simulink model "uc_faz_kompanzasyon"  (R2020b)
settings: Solver=VariableStepAuto  StartTime=0.0  StopTime=1  RelTol=1e-3  EnableMultiTasking=on
libraries: fl_lib x90, nesl_utility x45, powerlib_extras x15
settings Model: Creator=PC  LastModifiedBy=hilal
settings DataIOCC: ReturnWorkspaceOutputs=off
settings OptimizationCC: LifeSpan=inf
settings DebuggingCC: SFUnexpectedBacktrackingDiag=warning  SFNoUnconditionalDefaultTransitionDiag=warning  ArithmeticOperatorsInVariantConditions=warning
settings SFSimCC: SimUseLocalCustomCode=off  CustomCodeUndefinedFunction=UseInterfaceOnly
settings RTWCC: RTWUseLocalCustomCode=off
settings CodeAppCC: StateflowObjectComments=on
settings GRTTargetCC: TargetLangStandard=C89/C90 (ANSI)
settings ConfigComp: CovMetricSettings=dw  CovSaveCumulativeToWorkspaceVar=on  CovSaveSingleToWorkspaceVar=on  CovExternalEMLEnable=off
settings SimscapeCC: SimscapeNormalizeSystem=off

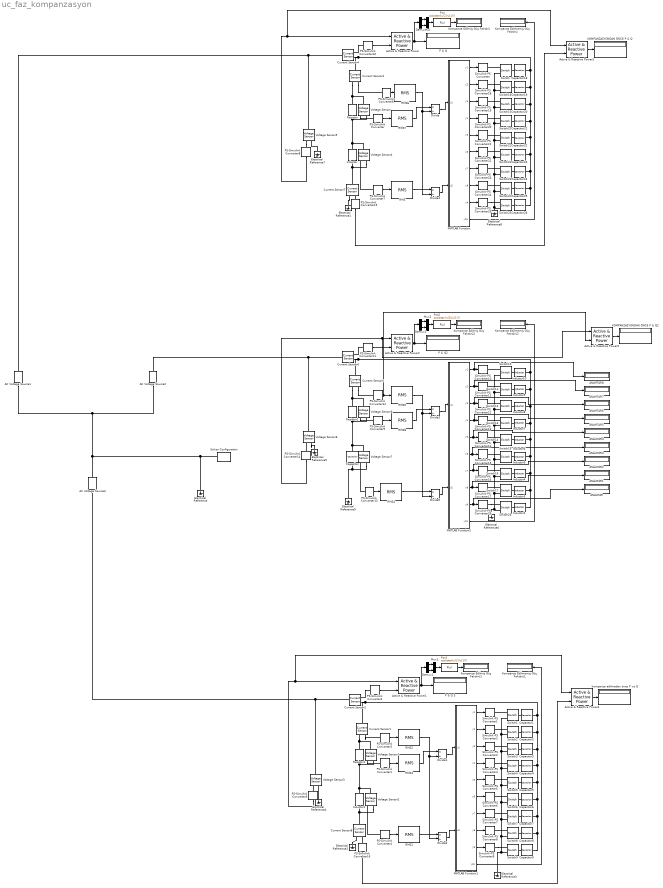
== system uc_faz_kompanzasyon ==
  AC Voltage Source1 : fl_lib/Electrical/Electrical Sources/AC Voltage Source  amp=200*sqrt(2) V  shift=0 rad  frequency=60 Hz  omega=50 Hz
  AC Voltage Source2 : fl_lib/Electrical/Electrical Sources/AC Voltage Source  amp=200*sqrt(2) V  shift=120 deg  frequency=60 Hz  omega=50 Hz
  AC Voltage Source3 : fl_lib/Electrical/Electrical Sources/AC Voltage Source  amp=200*sqrt(2) V  shift=240 deg  frequency=60 Hz  omega=50 Hz
  ANAHTAR{,1..8} (9 alike) : Display
  Active & Reactive Power{,1..5} (6 alike) : powerlib_extras/Measurements/Active & Reactive Power  f1=60
      settings: SourceProductBaseCode=PS
  Capacitor : fl_lib/Electrical/Electrical Elements/Capacitor  c=1/(20*2*pi*60) F  r=1e-6 Ohm  g=0 1/Ohm  i_specify=off  i_priority=None  i=0 A  i_nominal_specify=off  i_nominal_unit=A  i_nominal_value=1  v_specify=off  v_priority=None  v=0 V  v_nominal_specify=off  v_nominal_unit=V  v_nominal_value=1  vc_specify=off  vc_priority=High  vc=0 V  vc_nominal_specify=off  vc_nominal_unit=V  vc_nominal_value=1
  Capacitor1 : fl_lib/Electrical/Electrical Elements/Capacitor  c=5 uF  r=1e-6 Ohm  g=0 1/Ohm  i_specify=off  i_priority=None  i=0 A  i_nominal_specify=off  i_nominal_unit=A  i_nominal_value=1  v_specify=off  v_priority=None  v=0 V  v_nominal_specify=off  v_nominal_unit=V  v_nominal_value=1  vc_specify=off  vc_priority=High  vc=0 V  vc_nominal_specify=off  vc_nominal_unit=V  vc_nominal_value=1
  Capacitor18 : fl_lib/Electrical/Electrical Elements/Capacitor  c=6.319 uF  r=1e-6 Ohm  g=0 1/Ohm  i_specify=off  i_priority=None  i=0 A  i_nominal_specify=off  i_nominal_unit=A  i_nominal_value=1  v_specify=off  v_priority=None  v=0 V  v_nominal_specify=off  v_nominal_unit=V  v_nominal_value=1  vc_specify=off  vc_priority=High  vc=0 V  vc_nominal_specify=off  vc_nominal_unit=V  vc_nominal_value=1
  Capacitor19 : fl_lib/Electrical/Electrical Elements/Capacitor  c=15 uF  r=1e-6 Ohm  g=0 1/Ohm  i_specify=off  i_priority=None  i=0 A  i_nominal_specify=off  i_nominal_unit=A  i_nominal_value=1  v_specify=off  v_priority=None  v=0 V  v_nominal_specify=off  v_nominal_unit=V  v_nominal_value=1  vc_specify=off  vc_priority=High  vc=0 V  vc_nominal_specify=off  vc_nominal_unit=V  vc_nominal_value=1
  Capacitor2 : fl_lib/Electrical/Electrical Elements/Capacitor  c=15 uF  r=1e-6 Ohm  g=0 1/Ohm  i_specify=off  i_priority=None  i=0 A  i_nominal_specify=off  i_nominal_unit=A  i_nominal_value=1  v_specify=off  v_priority=None  v=0 V  v_nominal_specify=off  v_nominal_unit=V  v_nominal_value=1  vc_specify=off  vc_priority=High  vc=0 V  vc_nominal_specify=off  vc_nominal_unit=V  vc_nominal_value=1
  Capacitor20 : fl_lib/Electrical/Electrical Elements/Capacitor  c=24.6023 uF  r=1e-6 Ohm  g=0 1/Ohm  i_specify=off  i_priority=None  i=0 A  i_nominal_specify=off  i_nominal_unit=A  i_nominal_value=1  v_specify=off  v_priority=None  v=0 V  v_nominal_specify=off  v_nominal_unit=V  v_nominal_value=1  vc_specify=off  vc_priority=High  vc=0 V  vc_nominal_specify=off  vc_nominal_unit=V  vc_nominal_value=1
  Capacitor21 : fl_lib/Electrical/Electrical Elements/Capacitor  c=30.6 uF  r=1e-6 Ohm  g=0 1/Ohm  i_specify=off  i_priority=None  i=0 A  i_nominal_specify=off  i_nominal_unit=A  i_nominal_value=1  v_specify=off  v_priority=None  v=0 V  v_nominal_specify=off  v_nominal_unit=V  v_nominal_value=1  vc_specify=off  vc_priority=High  vc=0 V  vc_nominal_specify=off  vc_nominal_unit=V  vc_nominal_value=1
  Capacitor22 : fl_lib/Electrical/Electrical Elements/Capacitor  c=44.59 uF  r=1e-6 Ohm  g=0 1/Ohm  i_specify=off  i_priority=None  i=0 A  i_nominal_specify=off  i_nominal_unit=A  i_nominal_value=1  v_specify=off  v_priority=None  v=0 V  v_nominal_specify=off  v_nominal_unit=V  v_nominal_value=1  vc_specify=off  vc_priority=High  vc=0 V  vc_nominal_specify=off  vc_nominal_unit=V  vc_nominal_value=1
  Capacitor23 : fl_lib/Electrical/Electrical Elements/Capacitor  c=53.575 uF  r=1e-6 Ohm  g=0 1/Ohm  i_specify=off  i_priority=None  i=0 A  i_nominal_specify=off  i_nominal_unit=A  i_nominal_value=1  v_specify=off  v_priority=None  v=0 V  v_nominal_specify=off  v_nominal_unit=V  v_nominal_value=1  vc_specify=off  vc_priority=High  vc=0 V  vc_nominal_specify=off  vc_nominal_unit=V  vc_nominal_value=1
  Capacitor24 : fl_lib/Electrical/Electrical Elements/Capacitor  c=62.234 uF  r=1e-6 Ohm  g=0 1/Ohm  i_specify=off  i_priority=None  i=0 A  i_nominal_specify=off  i_nominal_unit=A  i_nominal_value=1  v_specify=off  v_priority=None  v=0 V  v_nominal_specify=off  v_nominal_unit=V  v_nominal_value=1  vc_specify=off  vc_priority=High  vc=0 V  vc_nominal_specify=off  vc_nominal_unit=V  vc_nominal_value=1
  Capacitor25 : fl_lib/Electrical/Electrical Elements/Capacitor  c=70.9489 uF  r=1e-6 Ohm  g=0 1/Ohm  i_specify=off  i_priority=None  i=0 A  i_nominal_specify=off  i_nominal_unit=A  i_nominal_value=1  v_specify=off  v_priority=None  v=0 V  v_nominal_specify=off  v_nominal_unit=V  v_nominal_value=1  vc_specify=off  vc_priority=High  vc=0 V  vc_nominal_specify=off  vc_nominal_unit=V  vc_nominal_value=1
  Capacitor26 : fl_lib/Electrical/Electrical Elements/Capacitor  c=78.304 uF  r=1e-6 Ohm  g=0 1/Ohm  i_specify=off  i_priority=None  i=0 A  i_nominal_specify=off  i_nominal_unit=A  i_nominal_value=1  v_specify=off  v_priority=None  v=0 V  v_nominal_specify=off  v_nominal_unit=V  v_nominal_value=1  vc_specify=off  vc_priority=High  vc=0 V  vc_nominal_specify=off  vc_nominal_unit=V  vc_nominal_value=1
  Capacitor3 : fl_lib/Electrical/Electrical Elements/Capacitor  c=24.6023 uF  r=1e-6 Ohm  g=0 1/Ohm  i_specify=off  i_priority=None  i=0 A  i_nominal_specify=off  i_nominal_unit=A  i_nominal_value=1  v_specify=off  v_priority=None  v=0 V  v_nominal_specify=off  v_nominal_unit=V  v_nominal_value=1  vc_specify=off  vc_priority=High  vc=0 V  vc_nominal_specify=off  vc_nominal_unit=V  vc_nominal_value=1
  Capacitor4 : fl_lib/Electrical/Electrical Elements/Capacitor  c=30.6 uF  r=1e-6 Ohm  g=0 1/Ohm  i_specify=off  i_priority=None  i=0 A  i_nominal_specify=off  i_nominal_unit=A  i_nominal_value=1  v_specify=off  v_priority=None  v=0 V  v_nominal_specify=off  v_nominal_unit=V  v_nominal_value=1  vc_specify=off  vc_priority=High  vc=0 V  vc_nominal_specify=off  vc_nominal_unit=V  vc_nominal_value=1
  Capacitor5 : fl_lib/Electrical/Electrical Elements/Capacitor  c=44.59 uF  r=1e-6 Ohm  g=0 1/Ohm  i_specify=off  i_priority=None  i=0 A  i_nominal_specify=off  i_nominal_unit=A  i_nominal_value=1  v_specify=off  v_priority=None  v=0 V  v_nominal_specify=off  v_nominal_unit=V  v_nominal_value=1  vc_specify=off  vc_priority=High  vc=0 V  vc_nominal_specify=off  vc_nominal_unit=V  vc_nominal_value=1
  Capacitor6 : fl_lib/Electrical/Electrical Elements/Capacitor  c=53.575 uF  r=1e-6 Ohm  g=0 1/Ohm  i_specify=off  i_priority=None  i=0 A  i_nominal_specify=off  i_nominal_unit=A  i_nominal_value=1  v_specify=off  v_priority=None  v=0 V  v_nominal_specify=off  v_nominal_unit=V  v_nominal_value=1  vc_specify=off  vc_priority=High  vc=0 V  vc_nominal_specify=off  vc_nominal_unit=V  vc_nominal_value=1
  Capacitor7 : fl_lib/Electrical/Electrical Elements/Capacitor  c=62.234 uF  r=1e-6 Ohm  g=0 1/Ohm  i_specify=off  i_priority=None  i=0 A  i_nominal_specify=off  i_nominal_unit=A  i_nominal_value=1  v_specify=off  v_priority=None  v=0 V  v_nominal_specify=off  v_nominal_unit=V  v_nominal_value=1  vc_specify=off  vc_priority=High  vc=0 V  vc_nominal_specify=off  vc_nominal_unit=V  vc_nominal_value=1
  Capacitor8 : fl_lib/Electrical/Electrical Elements/Capacitor  c=70.9489 uF  r=1e-6 Ohm  g=0 1/Ohm  i_specify=off  i_priority=None  i=0 A  i_nominal_specify=off  i_nominal_unit=A  i_nominal_value=1  v_specify=off  v_priority=None  v=0 V  v_nominal_specify=off  v_nominal_unit=V  v_nominal_value=1  vc_specify=off  vc_priority=High  vc=0 V  vc_nominal_specify=off  vc_nominal_unit=V  vc_nominal_value=1
  Capacitor9 : fl_lib/Electrical/Electrical Elements/Capacitor  c=78.304 uF  r=1e-6 Ohm  g=0 1/Ohm  i_specify=off  i_priority=None  i=0 A  i_nominal_specify=off  i_nominal_unit=A  i_nominal_value=1  v_specify=off  v_priority=None  v=0 V  v_nominal_specify=off  v_nominal_unit=V  v_nominal_value=1  vc_specify=off  vc_priority=High  vc=0 V  vc_nominal_specify=off  vc_nominal_unit=V  vc_nominal_value=1
  Current Sensor{1..8} (8 alike) : fl_lib/Electrical/Electrical Sensors/Current Sensor
  Demux : Demux  Outputs=2
  Demux1 : Demux  Outputs=2
  Demux2 : Demux  Outputs=2
  Divide{,1..5} (6 alike) : Product  Inputs=*/
  Electrical Reference{,1..9} (10 alike) : fl_lib/Electrical/Electrical Elements/Electrical Reference
  Fcn : Fcn  Expr=cos(atan(u(2)/u(1)))
  Fcn1 : Fcn  Expr=cos(atan(u(2)/u(1)))
  Fcn2 : Fcn  Expr=cos(atan(u(2)/u(1)))
  Inductor : fl_lib/Electrical/Electrical Elements/Inductor  l=20/(2*pi*60) H  r=0 Ohm  g=1e-9 1/Ohm  i_specify=off  i_priority=None  i=0 A  i_nominal_specify=off  i_nominal_unit=A  i_nominal_value=1  v_specify=off  v_priority=None  v=0 V  v_nominal_specify=off  v_nominal_unit=V  v_nominal_value=1  i_L_specify=off  i_L_priority=High  i_L=0 A  i_L_nominal_specify=off  i_L_nominal_unit=A  i_L_nominal_value=1
  Inductor1 : fl_lib/Electrical/Electrical Elements/Inductor  l=20/(2*pi*60) H  r=0 Ohm  g=1e-9 1/Ohm  i_specify=off  i_priority=None  i=0 A  i_nominal_specify=off  i_nominal_unit=A  i_nominal_value=1  v_specify=off  v_priority=None  v=0 V  v_nominal_specify=off  v_nominal_unit=V  v_nominal_value=1  i_L_specify=off  i_L_priority=High  i_L=0 A  i_L_nominal_specify=off  i_L_nominal_unit=A  i_L_nominal_value=1
  Inductor10 : fl_lib/Electrical/Electrical Elements/Inductor  l=1234 mH  r=0 Ohm  g=1e-9 1/Ohm  i_specify=off  i_priority=None  i=0 A  i_nominal_specify=off  i_nominal_unit=A  i_nominal_value=1  v_specify=off  v_priority=None  v=0 V  v_nominal_specify=off  v_nominal_unit=V  v_nominal_value=1  i_L_specify=off  i_L_priority=High  i_L=0 A  i_L_nominal_specify=off  i_L_nominal_unit=A  i_L_nominal_value=1
  Inductor2 : fl_lib/Electrical/Electrical Elements/Inductor  l=89.5 mH  r=0 Ohm  g=1e-9 1/Ohm  i_specify=off  i_priority=None  i=0 A  i_nominal_specify=off  i_nominal_unit=A  i_nominal_value=1  v_specify=off  v_priority=None  v=0 V  v_nominal_specify=off  v_nominal_unit=V  v_nominal_value=1  i_L_specify=off  i_L_priority=High  i_L=0 A  i_L_nominal_specify=off  i_L_nominal_unit=A  i_L_nominal_value=1
  Inductor3 : fl_lib/Electrical/Electrical Elements/Inductor  l=99 mH  r=0 Ohm  g=1e-9 1/Ohm  i_specify=off  i_priority=None  i=0 A  i_nominal_specify=off  i_nominal_unit=A  i_nominal_value=1  v_specify=off  v_priority=None  v=0 V  v_nominal_specify=off  v_nominal_unit=V  v_nominal_value=1  i_L_specify=off  i_L_priority=High  i_L=0 A  i_L_nominal_specify=off  i_L_nominal_unit=A  i_L_nominal_value=1
  Inductor4 : fl_lib/Electrical/Electrical Elements/Inductor  l=109.9 mH  r=0 Ohm  g=1e-9 1/Ohm  i_specify=off  i_priority=None  i=0 A  i_nominal_specify=off  i_nominal_unit=A  i_nominal_value=1  v_specify=off  v_priority=None  v=0 V  v_nominal_specify=off  v_nominal_unit=V  v_nominal_value=1  i_L_specify=off  i_L_priority=High  i_L=0 A  i_L_nominal_specify=off  i_L_nominal_unit=A  i_L_nominal_value=1
  Inductor5 : fl_lib/Electrical/Electrical Elements/Inductor  l=136 mH  r=0 Ohm  g=1e-9 1/Ohm  i_specify=off  i_priority=None  i=0 A  i_nominal_specify=off  i_nominal_unit=A  i_nominal_value=1  v_specify=off  v_priority=None  v=0 V  v_nominal_specify=off  v_nominal_unit=V  v_nominal_value=1  i_L_specify=off  i_L_priority=High  i_L=0 A  i_L_nominal_specify=off  i_L_nominal_unit=A  i_L_nominal_value=1
  Inductor6 : fl_lib/Electrical/Electrical Elements/Inductor  l=158 mH  r=0 Ohm  g=1e-9 1/Ohm  i_specify=off  i_priority=None  i=0 A  i_nominal_specify=off  i_nominal_unit=A  i_nominal_value=1  v_specify=off  v_priority=None  v=0 V  v_nominal_specify=off  v_nominal_unit=V  v_nominal_value=1  i_L_specify=off  i_L_priority=High  i_L=0 A  i_L_nominal_specify=off  i_L_nominal_unit=A  i_L_nominal_value=1
  Inductor7 : fl_lib/Electrical/Electrical Elements/Inductor  l=210 mH  r=0 Ohm  g=1e-9 1/Ohm  i_specify=off  i_priority=None  i=0 A  i_nominal_specify=off  i_nominal_unit=A  i_nominal_value=1  v_specify=off  v_priority=None  v=0 V  v_nominal_specify=off  v_nominal_unit=V  v_nominal_value=1  i_L_specify=off  i_L_priority=High  i_L=0 A  i_L_nominal_specify=off  i_L_nominal_unit=A  i_L_nominal_value=1
  Inductor8 : fl_lib/Electrical/Electrical Elements/Inductor  l=269 mH  r=0 Ohm  g=1e-9 1/Ohm  i_specify=off  i_priority=None  i=0 A  i_nominal_specify=off  i_nominal_unit=A  i_nominal_value=1  v_specify=off  v_priority=None  v=0 V  v_nominal_specify=off  v_nominal_unit=V  v_nominal_value=1  i_L_specify=off  i_L_priority=High  i_L=0 A  i_L_nominal_specify=off  i_L_nominal_unit=A  i_L_nominal_value=1
  Inductor9 : fl_lib/Electrical/Electrical Elements/Inductor  l=508 mH  r=0 Ohm  g=1e-9 1/Ohm  i_specify=off  i_priority=None  i=0 A  i_nominal_specify=off  i_nominal_unit=A  i_nominal_value=1  v_specify=off  v_priority=None  v=0 V  v_nominal_specify=off  v_nominal_unit=V  v_nominal_value=1  i_L_specify=off  i_L_priority=High  i_L=0 A  i_L_nominal_specify=off  i_L_nominal_unit=A  i_L_nominal_value=1
  KOMPANZASYONDAN ÖNCE P & Q : Display
  KOMPANZASYONDAN ÖNCE P & Q2 : Display
  Kompanze Edilmemiş Güç Faktörü : Display
  Kompanze Edilmemiş Güç Faktörü1 : Display
  Kompanze Edilmemiş Güç Faktörü2 : Display
  Kompanze Edilmiş Güç Faktörü : Display
  Kompanze Edilmiş Güç Faktörü1 : Display
  Kompanze Edilmiş Güç Faktörü2 : Display
  MATLAB Function : MATLAB Function  TreatAsAtomicUnit=on
  MATLAB Function1 : MATLAB Function  TreatAsAtomicUnit=on
  MATLAB Function2 : MATLAB Function  TreatAsAtomicUnit=on
  Mux : Mux  Inputs=2
  Mux1 : Mux  Inputs=2
  Mux2 : Mux  Inputs=2
  P & Q : Display
  P & Q 3 : Display
  P & Q2 : Display
  PS-Simulink Converter{,1..16} (17 alike) : nesl_utility/PS-Simulink Converter  PhysicalDomain=network_engine_domain  SubClassName=ps_output  LeftPortType=input  RightPortType=output  PseudoPeriodic=off  Frequencies=[]  Unit=1  AffineConversion=off
  RMS{,1..8} (9 alike) : powerlib_extras/Measurements/RMS  f1=60
      settings: SourceProductBaseCode=PS
  Resistor : fl_lib/Electrical/Electrical Elements/Resistor  R=45 Ohm  i_specify=off  i_priority=None  i=0 A  i_nominal_specify=off  i_nominal_unit=A  i_nominal_value=1  v_specify=off  v_priority=None  v=0 V  v_nominal_specify=off  v_nominal_unit=V  v_nominal_value=1
  Resistor1 : fl_lib/Electrical/Electrical Elements/Resistor  R=13.5 Ohm  i_specify=off  i_priority=None  i=0 A  i_nominal_specify=off  i_nominal_unit=A  i_nominal_value=1  v_specify=off  v_priority=None  v=0 V  v_nominal_specify=off  v_nominal_unit=V  v_nominal_value=1
  Resistor2 : fl_lib/Electrical/Electrical Elements/Resistor  R=20 Ohm  i_specify=off  i_priority=None  i=0 A  i_nominal_specify=off  i_nominal_unit=A  i_nominal_value=1  v_specify=off  v_priority=None  v=0 V  v_nominal_specify=off  v_nominal_unit=V  v_nominal_value=1
  Simulink-PS Converter{,1..26} (27 alike) : nesl_utility/Simulink-PS Converter  PhysicalDomain=network_engine_domain  SubClassName=ps_input  LeftPortType=input  RightPortType=output  PseudoPeriodic=off  Frequencies=[]  NoiseDistribution=none  NoiseParameters=[]  Unit=1  AffineConversion=off  FilteringAndDerivatives=zero  SimscapeFilterOrder=1  InputFilterTimeConstant=0.001  UdotUserProvided=1
  Solver Configuration : nesl_utility/Solver Configuration  PhysicalDomain=network_engine_domain  SubClassName=solver  LeftPortType=input  RightPortType=generic  Tones=[]  Harmonics=[]  SimulateNoise=off  Profile=off  UseLocalSampling=off  EnableSwitchedLinearOptims=on  FrequencyDomain=off  UseCCode=off  RelTol=0.001  AbsTol=1e-06  MinStep=1e-09  ToWorkspace=off  RevertToSquareIcSolve=off  NumHomotopyIterations=100  PhasorMode=off  PhasorModeNumHarmonics=1  DoDC=on  ResidualTolerance=1e-9  UseLocalSolver=off  LocalSolverChoice=NE_BACKWARD_EULER_ADVANCER  LocalSolverSampleTime=.001  DoFixedCost=off  MaxNonlinIter=3  MaxModeIter=2  ComputeImpulses=off  ImpulseIterations=2  LinearAlgebra=Sparse  EquationFormulation=NE_TIME_EF  DelaysMemoryBudget=1024  AutomaticFiltering=on  FilteringTimeConstant=0.001  PartitionStorageMethod=AS_NEEDED  PartitionMemoryBudget=1024  PartitionMethod=FAST
  Switch{,1..26} (27 alike) : fl_lib/Electrical/Electrical Elements/Switch  R_closed=0.01 Ohm  G_open=1e-8 1/Ohm  Threshold=0  i_specify=off  i_priority=None  i=0 A  i_nominal_specify=off  i_nominal_unit=A  i_nominal_value=1  v_specify=off  v_priority=None  v=0 V  v_nominal_specify=off  v_nominal_unit=V  v_nominal_value=1
  Voltage Sensor{,1..8} (9 alike) : fl_lib/Electrical/Electrical Sensors/Voltage Sensor
  kompanze edilmeden önce P ve Q : Display
  wires:
  MATLAB Function/1(y1) -> Simulink-PS Converter/1
  MATLAB Function/3(y3) -> Simulink-PS Converter19/1
  MATLAB Function/5(y5) -> Simulink-PS Converter21/1
  MATLAB Function/7(y7) -> Simulink-PS Converter23/1
  MATLAB Function/8(y8) -> Simulink-PS Converter24/1
  MATLAB Function/6(y6) -> Simulink-PS Converter22/1
  Divide/1 -> MATLAB Function/1(u1)
  MATLAB Function/9(y9) -> Simulink-PS Converter25/1
  PS-Simulink Converter6/1 -> RMS6/1
  PS-Simulink Converter/1 -> RMS7/1
  PS-Simulink Converter7/1 -> RMS/1
  RMS/1 -> Divide4/1
  RMS6/1 -> Divide/2, Divide4/2
  RMS7/1 -> Divide/1
  Active & Reactive Power/1 -> P & Q/1, Demux/1
  Divide4/1 -> MATLAB Function/2(u2)
  PS-Simulink Converter10/1 -> Active & Reactive Power/2
  MATLAB Function/10(y10) -> Kompanze Edilmemiş Güç Faktörü/1
  Demux/1 -> Mux/1
  Demux/2 -> Mux/2
  Mux/1 -> Fcn/1
  Fcn/1 -> Kompanze Edilmiş Güç Faktörü/1
  MATLAB Function1/1(y1) -> Simulink-PS Converter1/1
  MATLAB Function1/2(y2) -> Simulink-PS Converter2/1
  MATLAB Function1/3(y3) -> Simulink-PS Converter3/1
  MATLAB Function1/4(y4) -> Simulink-PS Converter4/1
  MATLAB Function1/5(y5) -> Simulink-PS Converter5/1
  MATLAB Function1/7(y7) -> Simulink-PS Converter7/1
  MATLAB Function1/8(y8) -> Simulink-PS Converter8/1
  MATLAB Function1/6(y6) -> Simulink-PS Converter6/1
  Divide1/1 -> MATLAB Function1/1(u1)
  PS-Simulink Converter3/1 -> RMS2/1
  PS-Simulink Converter1/1 -> RMS3/1
  PS-Simulink Converter4/1 -> RMS1/1
  RMS1/1 -> Divide2/1
  RMS2/1 -> Divide1/2, Divide2/2
  RMS3/1 -> Divide1/1
  Active & Reactive Power1/1 -> P & Q 3/1, Demux1/1
  PS-Simulink Converter5/1 -> Active & Reactive Power4/1, Active & Reactive Power1/1
  Divide2/1 -> MATLAB Function1/2(u2)
  PS-Simulink Converter2/1 -> Active & Reactive Power1/2
  MATLAB Function1/10(y10) -> Kompanze Edilmemiş Güç Faktörü1/1
  Demux1/1 -> Mux1/1
  Demux1/2 -> Mux1/2
  Mux1/1 -> Fcn1/1
  Fcn1/1 -> Kompanze Edilmiş Güç Faktörü1/1
  MATLAB Function2/1(y1) -> ANAHTAR8/1, Simulink-PS Converter10/1
  MATLAB Function2/2(y2) -> ANAHTAR7/1, Simulink-PS Converter11/1
  MATLAB Function2/3(y3) -> ANAHTAR6/1, Simulink-PS Converter12/1
  MATLAB Function2/4(y4) -> ANAHTAR5/1, Simulink-PS Converter13/1
  MATLAB Function2/5(y5) -> ANAHTAR4/1, Simulink-PS Converter14/1
  MATLAB Function2/7(y7) -> ANAHTAR2/1, Simulink-PS Converter16/1
  MATLAB Function2/8(y8) -> ANAHTAR1/1, Simulink-PS Converter17/1
  MATLAB Function2/6(y6) -> ANAHTAR3/1, Simulink-PS Converter15/1
  Divide3/1 -> MATLAB Function2/1(u1)
  MATLAB Function2/9(y9) -> ANAHTAR/1, Simulink-PS Converter26/1
  PS-Simulink Converter12/1 -> Active & Reactive Power5/2, RMS5/1
  PS-Simulink Converter9/1 -> RMS8/1
  PS-Simulink Converter13/1 -> RMS4/1
  RMS5/1 -> Divide3/2, Divide5/2
  RMS8/1 -> Divide3/1
  Active & Reactive Power2/1 -> P & Q2/1, Demux2/1
  PS-Simulink Converter14/1 -> Active & Reactive Power5/1, Active & Reactive Power2/1
  Divide5/1 -> MATLAB Function2/2(u2)
  PS-Simulink Converter11/1 -> Active & Reactive Power2/2
  MATLAB Function2/10(y10) -> Kompanze Edilmemiş Güç Faktörü2/1
  Demux2/1 -> Mux2/1
  Demux2/2 -> Mux2/2
  Mux2/1 -> Fcn2/1
  Fcn2/1 -> Kompanze Edilmiş Güç Faktörü2/1
  RMS4/1 -> Divide5/1
  MATLAB Function/2(y2) -> Simulink-PS Converter18/1
  MATLAB Function/4(y4) -> Simulink-PS Converter20/1
  Active & Reactive Power3/1 -> KOMPANZASYONDAN ÖNCE P & Q/1
  PS-Simulink Converter8/1 -> Active & Reactive Power3/1, Active & Reactive Power/1
  PS-Simulink Converter15/1 -> Active & Reactive Power3/2
  Active & Reactive Power4/1 -> kompanze edilmeden önce P ve Q/1
  PS-Simulink Converter16/1 -> Active & Reactive Power4/2
  MATLAB Function1/9(y9) -> Simulink-PS Converter9/1
  Active & Reactive Power5/1 -> KOMPANZASYONDAN ÖNCE P & Q2/1
  connections:
  Capacitor21/RConn1 -- Current Sensor3/LConn1 -- Current Sensor4/RConn2 -- Capacitor18/RConn1 -- Capacitor19/RConn1 -- Capacitor20/RConn1 -- Capacitor26/RConn1 -- Capacitor25/RConn1 -- Capacitor24/RConn1 -- Capacitor23/RConn1 -- Capacitor22/RConn1
  Resistor/RConn1 -- Voltage Sensor/RConn2 -- Voltage Sensor4/LConn1 -- Inductor/LConn1
  Voltage Sensor/LConn1 -- Resistor/LConn1 -- Current Sensor3/RConn2
  Current Sensor4/LConn1 -- Voltage Sensor5/LConn1 -- AC Voltage Source1/LConn1
  Capacitor19/LConn1 -- Switch18/LConn1
  Capacitor20/LConn1 -- Switch19/LConn1
  Capacitor21/LConn1 -- Switch20/LConn1
  Switch23/RConn1 -- Simulink-PS Converter23/RConn1
  Capacitor24/LConn1 -- Switch23/LConn1
  Voltage Sensor/RConn1 -- PS-Simulink Converter/LConn1
  Capacitor25/LConn1 -- Switch24/LConn1
  Simulink-PS Converter25/RConn1 -- Switch25/RConn1
  Switch20/RConn1 -- Simulink-PS Converter20/RConn1
  Capacitor26/LConn1 -- Switch25/LConn1
  Switch19/RConn1 -- Simulink-PS Converter19/RConn1
  Switch22/RConn1 -- Simulink-PS Converter22/RConn1
  Capacitor18/LConn1 -- Switch/LConn1
  Switch/RConn1 -- Simulink-PS Converter/RConn1
  Capacitor22/LConn1 -- Switch21/LConn1
  Capacitor23/LConn1 -- Switch22/LConn1
  Voltage Sensor5/RConn1 -- PS-Simulink Converter8/LConn1
  Switch18/RConn1 -- Simulink-PS Converter18/RConn1
  PS-Simulink Converter7/LConn1 -- Voltage Sensor4/RConn1
  Current Sensor4/RConn1 -- PS-Simulink Converter10/LConn1
  Switch21/RConn1 -- Simulink-PS Converter21/RConn1
  Switch24/RConn1 -- Simulink-PS Converter24/RConn1
  Capacitor4/RConn1 -- Current Sensor1/LConn1 -- Current Sensor2/RConn2 -- Capacitor1/RConn1 -- Capacitor2/RConn1 -- Capacitor3/RConn1 -- Capacitor5/RConn1 -- Capacitor6/RConn1 -- Capacitor7/RConn1 -- Capacitor9/RConn1 -- Capacitor8/RConn1
  AC Voltage Source2/RConn1 -- AC Voltage Source1/RConn1 -- Electrical Reference/LConn1 -- Solver Configuration/RConn1 -- AC Voltage Source3/RConn1
  Inductor1/LConn1 -- Voltage Sensor2/LConn1 -- Voltage Sensor1/RConn2 -- Resistor1/RConn1
  Voltage Sensor1/LConn1 -- Resistor1/LConn1 -- Current Sensor1/RConn2
  Current Sensor2/LConn1 -- Voltage Sensor3/LConn1 -- AC Voltage Source3/LConn1
  Voltage Sensor1/RConn1 -- PS-Simulink Converter1/LConn1
  Capacitor2/LConn1 -- Switch2/LConn1
  Capacitor4/LConn1 -- Switch4/LConn1
  Current Sensor1/RConn1 -- PS-Simulink Converter3/LConn1
  PS-Simulink Converter4/LConn1 -- Voltage Sensor2/RConn1
  Capacitor8/LConn1 -- Switch8/LConn1
  Capacitor6/LConn1 -- Switch6/LConn1
  Switch3/RConn1 -- Simulink-PS Converter3/RConn1
  Switch6/RConn1 -- Simulink-PS Converter6/RConn1
  Switch1/RConn1 -- Simulink-PS Converter1/RConn1
  Switch5/RConn1 -- Simulink-PS Converter5/RConn1
  Capacitor9/LConn1 -- Switch9/LConn1
  Switch8/RConn1 -- Simulink-PS Converter8/RConn1
  Capacitor7/LConn1 -- Switch7/LConn1
  Simulink-PS Converter9/RConn1 -- Switch9/RConn1
  Switch7/RConn1 -- Simulink-PS Converter7/RConn1
  Capacitor3/LConn1 -- Switch3/LConn1
  Capacitor1/LConn1 -- Switch1/LConn1
  Switch4/RConn1 -- Simulink-PS Converter4/RConn1
  Current Sensor2/RConn1 -- PS-Simulink Converter2/LConn1
  Switch2/RConn1 -- Simulink-PS Converter2/RConn1
  Capacitor5/LConn1 -- Switch5/LConn1
  Inductor7/RConn1 -- Inductor6/RConn1 -- Inductor5/RConn1 -- Inductor4/RConn1 -- Inductor3/RConn1 -- Inductor2/RConn1 -- Inductor9/RConn1 -- Inductor10/RConn1 -- Current Sensor5/LConn1 -- Current Sensor6/RConn2 -- Inductor8/RConn1
  Voltage Sensor7/LConn1 -- Capacitor/LConn1 -- Voltage Sensor6/RConn2 -- Resistor2/RConn1
  Voltage Sensor6/LConn1 -- Resistor2/LConn1 -- Current Sensor5/RConn2
  Inductor4/LConn1 -- Switch16/LConn1
  Switch13/RConn1 -- Simulink-PS Converter13/RConn1
  Inductor10/LConn1 -- Switch10/LConn1
  Switch11/RConn1 -- Simulink-PS Converter11/RConn1
  Switch10/RConn1 -- Simulink-PS Converter10/RConn1
  Switch12/RConn1 -- Simulink-PS Converter12/RConn1
  Voltage Sensor6/RConn1 -- PS-Simulink Converter9/LConn1
  Inductor9/LConn1 -- Switch11/LConn1
  Switch14/RConn1 -- Simulink-PS Converter14/RConn1
  Current Sensor6/RConn1 -- PS-Simulink Converter11/LConn1
  Inductor8/LConn1 -- Switch12/LConn1
  Inductor3/LConn1 -- Switch17/LConn1
  Current Sensor5/RConn1 -- PS-Simulink Converter12/LConn1
  Inductor2/LConn1 -- Switch26/LConn1
  Switch15/RConn1 -- Simulink-PS Converter15/RConn1
  Switch16/RConn1 -- Simulink-PS Converter16/RConn1
  Inductor7/LConn1 -- Switch13/LConn1
  Inductor5/LConn1 -- Switch15/LConn1
  Inductor6/LConn1 -- Switch14/LConn1
  Switch17/RConn1 -- Simulink-PS Converter17/RConn1
  Simulink-PS Converter26/RConn1 -- Switch26/RConn1
  PS-Simulink Converter13/LConn1 -- Voltage Sensor7/RConn1
  PS-Simulink Converter14/LConn1 -- Voltage Sensor8/RConn1
  AC Voltage Source2/LConn1 -- Current Sensor6/LConn1 -- Voltage Sensor8/LConn1
  Current Sensor3/RConn1 -- PS-Simulink Converter6/LConn1
  Voltage Sensor4/RConn2 -- Inductor/RConn1 -- Current Sensor7/LConn1
  PS-Simulink Converter15/LConn1 -- Current Sensor7/RConn1
  Current Sensor7/RConn2 -- Electrical Reference1/LConn1
  Voltage Sensor2/RConn2 -- Inductor1/RConn1 -- Current Sensor8/LConn1
  Current Sensor8/RConn2 -- Electrical Reference2/LConn1
  PS-Simulink Converter16/LConn1 -- Current Sensor8/RConn1
  PS-Simulink Converter5/LConn1 -- Voltage Sensor3/RConn1
  Switch9/RConn2 -- Electrical Reference3/LConn1 -- Switch4/RConn2 -- Switch3/RConn2 -- Switch1/RConn2 -- Switch2/RConn2 -- Switch5/RConn2 -- Switch6/RConn2 -- Switch7/RConn2 -- Switch8/RConn2
  Electrical Reference4/LConn1 -- Voltage Sensor3/RConn2
  Voltage Sensor8/RConn2 -- Electrical Reference5/LConn1
  Switch17/RConn2 -- Electrical Reference6/LConn1 -- Switch26/RConn2 -- Switch13/RConn2 -- Switch12/RConn2 -- Switch10/RConn2 -- Switch11/RConn2 -- Switch14/RConn2 -- Switch15/RConn2 -- Switch16/RConn2
  Electrical Reference7/LConn1 -- Voltage Sensor5/RConn2
  Switch23/RConn2 -- Electrical Reference8/LConn1 -- Switch25/RConn2 -- Switch24/RConn2 -- Switch20/RConn2 -- Switch19/RConn2 -- Switch/RConn2 -- Switch18/RConn2 -- Switch21/RConn2 -- Switch22/RConn2
  Voltage Sensor7/RConn2 -- Electrical Reference9/LConn1 -- Capacitor/RConn1

== matlab function uc_faz_kompanzasyon/MATLAB Function1 ==
  data: u1 input; y1 output; u2 input; y2 output; y3 output; y4 output; y5 output; y6 output; y7 output; y8 output; y9 output; y10 output
function [y1,y2,y3,y4,y5,y6,y7,y8,y9,y10] = fcn(u1,u2)
R=u1;% 1. değişken
L=u2;% 1. değişken

V=200;

I=200/(R+i*L);
Iconj=conj(I);

S=V*Iconj;
P=real(S);
Q=imag(S);

teta=angle(S);
pf=cos(teta);

if(pf>=0.9 && pf<=0.95)
    y1=1;
    y2=0;
    y3=0;
    y4=0;
    y5=0;
    y6=0;
    y7=0;
    y8=0;
    y9=0;
    y10=pf;
elseif(pf>=0.85 && pf<=0.9)
    y1=0;
    y2=1;
    y3=0;
    y4=0;
    y5=0;
    y6=0;
    y7=0;
    y8=0;
    y9=0;
    y10=pf;
elseif(pf>=0.80 && pf<=0.85)
    y1=0;
    y2=0;
    y3=1;
    y4=0;
    y5=0;
    y6=0;
    y7=0;
    y8=0;
    y9=0;
    y10=pf;
elseif(pf>=0.75 && pf<=0.80)
    y1=0;
    y2=0;
    y3=0;
    y4=1;
    y5=0;
    y6=0;
    y7=0;
    y8=0;
    y9=0;
    y10=pf;
elseif(pf>=0.70 && pf<=0.75)
    y1=0;
    y2=0;
    y3=0;
    y4=0;
    y5=1;
    y6=0;
    y7=0;
    y8=0;
    y9=0;
    y10=pf;
elseif(pf>=0.65 && pf<=0.70)
    y1=0;
    y2=0;
    y3=0;
    y4=0;
    y5=0;
    y6=1;
    y7=0;
    y8=0;
    y9=0;
    y10=pf;
elseif(pf>=0.60 && pf<=0.65)
    y1=0;
    y2=0;
    y3=0;
    y4=0;
    y5=0;
    y6=0;
    y7=1;
    y8=0;
    y9=0;
    y10=pf;
elseif(pf>=0.55 && pf<=0.60)
    y1=0;
    y2=0;
    y3=0;
    y4=0;
    y5=0;
    y6=0;
    y7=0;
    y8=1;
    y9=0;
    y10=pf;
elseif(pf>=0.50 && pf<=0.55)
    y1=0;
    y2=0;
    y3=0;
    y4=0;
    y5=0;
    y6=0;
    y7=0;
    y8=0;
    y9=1;
    y10=pf;
else
    y1=0;
    y2=0;
    y3=0;
    y4=0;
    y5=0;
    y6=0;
    y7=0;
    y8=0;
    y9=0;
    y10=pf;
    
end

== matlab function uc_faz_kompanzasyon/MATLAB Function2 ==
  data: u1 input; y1 output; u2 input; y2 output; y3 output; y4 output; y5 output; y6 output; y7 output; y8 output; y9 output; y10 output
function [y1,y2,y3,y4,y5,y6,y7,y8,y9,y10] = fcn(u1,u2)
R=u1;% 1. değişken
C=u2;% 1. değişken

V=200;

I=200/(R-i*C);
Iconj=conj(I);

S=V*Iconj;
P=real(S);
Q=imag(S);

teta=angle(S);
pf=cos(teta);

if(pf>=0.9 && pf<=0.95)
    y1=1;
    y2=0;
    y3=0;
    y4=0;
    y5=0;
    y6=0;
    y7=0;
    y8=0;
    y9=0;
    y10=pf;
elseif(pf>=0.85 && pf<=0.9)
    y1=0;
    y2=1;
    y3=0;
    y4=0;
    y5=0;
    y6=0;
    y7=0;
    y8=0;
    y9=0;
    y10=pf;
elseif(pf>=0.80 && pf<=0.85)
    y1=0;
    y2=0;
    y3=1;
    y4=0;
    y5=0;
    y6=0;
    y7=0;
    y8=0;
    y9=0;
    y10=pf;
elseif(pf>=0.75 && pf<=0.80)
    y1=0;
    y2=0;
    y3=0;
    y4=1;
    y5=0;
    y6=0;
    y7=0;
    y8=0;
    y9=0;
    y10=pf;
elseif(pf>=0.70 && pf<=0.75)
    y1=0;
    y2=0;
    y3=0;
    y4=0;
    y5=1;
    y6=0;
    y7=0;
    y8=0;
    y9=0;
    y10=pf;
elseif(pf>=0.65 && pf<=0.70)
    y1=0;
    y2=0;
    y3=0;
    y4=0;
    y5=0;
    y6=1;
    y7=0;
    y8=0;
    y9=0;
    y10=pf;
elseif(pf>=0.60 && pf<=0.65)
    y1=0;
    y2=0;
    y3=0;
    y4=0;
    y5=0;
    y6=0;
    y7=1;
    y8=0;
    y9=0;
    y10=pf;
elseif(pf>=0.55 && pf<=0.60)
    y1=0;
    y2=0;
    y3=0;
    y4=0;
    y5=0;
    y6=0;
    y7=0;
    y8=1;
    y9=0;
    y10=pf;
elseif(pf>=0.50 && pf<=0.55)
    y1=0;
    y2=0;
    y3=0;
    y4=0;
    y5=0;
    y6=0;
    y7=0;
    y8=0;
    y9=1;
    y10=pf;
else
    y1=0;
    y2=0;
    y3=0;
    y4=0;
    y5=0;
    y6=0;
    y7=0;
    y8=0;
    y9=0;
    y10=pf;
    
end

== matlab function uc_faz_kompanzasyon/MATLAB Function ==
  data: u1 input; y1 output; u2 input; y2 output; y3 output; y4 output; y5 output; y6 output; y7 output; y8 output; y9 output; y10 output
function [y1,y2,y3,y4,y5,y6,y7,y8,y9,y10] = fcn(u1,u2)
R=u1;% 1. değişken
L=u2;% 1. değişken

V=200;

I=200/(R+i*L);
Iconj=conj(I);

S=V*Iconj;
P=real(S);
Q=imag(S);

teta=angle(S);
pf=cos(teta);

if(pf>=0.9 && pf<=0.95)
    y1=1;
    y2=0;
    y3=0;
    y4=0;
    y5=0;
    y6=0;
    y7=0;
    y8=0;
    y9=0;
    y10=pf;
elseif(pf>=0.85 && pf<=0.9)
    y1=0;
    y2=1;
    y3=0;
    y4=0;
    y5=0;
    y6=0;
    y7=0;
    y8=0;
    y9=0;
    y10=pf;
elseif(pf>=0.80 && pf<=0.85)
    y1=0;
    y2=0;
    y3=1;
    y4=0;
    y5=0;
    y6=0;
    y7=0;
    y8=0;
    y9=0;
    y10=pf;
elseif(pf>=0.75 && pf<=0.80)
    y1=0;
    y2=0;
    y3=0;
    y4=1;
    y5=0;
    y6=0;
    y7=0;
    y8=0;
    y9=0;
    y10=pf;
elseif(pf>=0.70 && pf<=0.75)
    y1=0;
    y2=0;
    y3=0;
    y4=0;
    y5=1;
    y6=0;
    y7=0;
    y8=0;
    y9=0;
    y10=pf;
elseif(pf>=0.65 && pf<=0.70)
    y1=0;
    y2=0;
    y3=0;
    y4=0;
    y5=0;
    y6=1;
    y7=0;
    y8=0;
    y9=0;
    y10=pf;
elseif(pf>=0.60 && pf<=0.65)
    y1=0;
    y2=0;
    y3=0;
    y4=0;
    y5=0;
    y6=0;
    y7=1;
    y8=0;
    y9=0;
    y10=pf;
elseif(pf>=0.55 && pf<=0.60)
    y1=0;
    y2=0;
    y3=0;
    y4=0;
    y5=0;
    y6=0;
    y7=0;
    y8=1;
    y9=0;
    y10=pf;
elseif(pf>=0.50 && pf<=0.55)
    y1=0;
    y2=0;
    y3=0;
    y4=0;
    y5=0;
    y6=0;
    y7=0;
    y8=0;
    y9=1;
    y10=pf;
else
    y1=0;
    y2=0;
    y3=0;
    y4=0;
    y5=0;
    y6=0;
    y7=0;
    y8=0;
    y9=0;
    y10=pf;
    
end
